simulink model "signalProcess"  (R2016a)
settings: Solver=VariableStepAuto  StartTime=0.0  StopTime=10  RelTol=1e-3
libraries: powerlib x11, powerlib_meascontrol x1
settings Model: Creator=Jasonkay  LastModifiedBy=Jasonkay

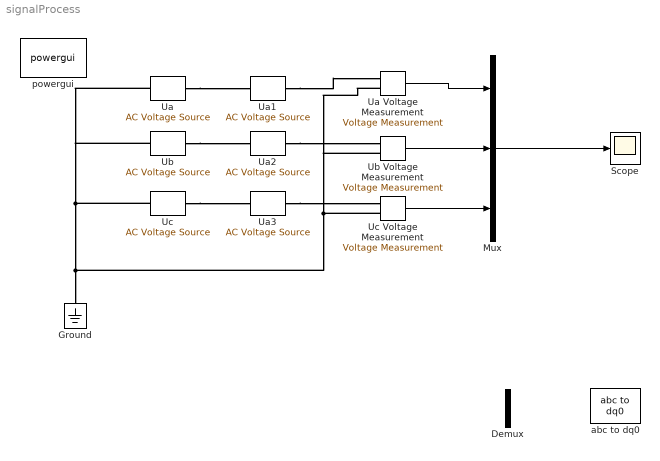
== system signalProcess ==
  Demux : Demux  Outputs=2
  Ground : powerlib/Elements/Ground  LConnTagsString=a
  Mux : Mux  Inputs=3
  Scope : Scope
  Ua : powerlib/Electrical Sources/AC Voltage Source  Amplitude=220 * sqrt(2)  Phase=0  Frequency=50  SampleTime=0  Measurements=None  BusType=swing  Pref=10e3  Qref=0  Qmin=-inf  Qmax=+inf
  Ua Voltage Measurement : powerlib/Measurements/Voltage Measurement  PhasorSimulation=off  OutputType=Complex  PSBequivalent=0
  Ua1 : powerlib/Electrical Sources/AC Voltage Source  Amplitude=20 * sqrt(2)  Phase=0  Frequency=50.1  SampleTime=0  Measurements=None  BusType=swing  Pref=10e3  Qref=0  Qmin=-inf  Qmax=+inf
  Ua2 : powerlib/Electrical Sources/AC Voltage Source  Amplitude=20 * sqrt(2)  Phase=0  Frequency=50.1  SampleTime=0  Measurements=None  BusType=swing  Pref=10e3  Qref=0  Qmin=-inf  Qmax=+inf
  Ua3 : powerlib/Electrical Sources/AC Voltage Source  Amplitude=20 * sqrt(2)  Phase=0  Frequency=50.1  SampleTime=0  Measurements=None  BusType=swing  Pref=10e3  Qref=0  Qmin=-inf  Qmax=+inf
  Ub : powerlib/Electrical Sources/AC Voltage Source  Amplitude=220 * sqrt(2)  Phase=240  Frequency=50  SampleTime=0  Measurements=None  BusType=swing  Pref=10e3  Qref=0  Qmin=-inf  Qmax=+inf
  Ub Voltage Measurement : powerlib/Measurements/Voltage Measurement  PhasorSimulation=off  OutputType=Complex  PSBequivalent=0
  Uc : powerlib/Electrical Sources/AC Voltage Source  Amplitude=220 * sqrt(2)  Phase=120  Frequency=50  SampleTime=0  Measurements=None  BusType=swing  Pref=10e3  Qref=0  Qmin=-inf  Qmax=+inf
  Uc Voltage Measurement : powerlib/Measurements/Voltage Measurement  PhasorSimulation=off  OutputType=Complex  PSBequivalent=0
  abc to dq0 : powerlib_meascontrol/Transformations/abc to dq0  Alignment=90 degrees behind phase A axis
  powergui : powerlib/powergui  Priority=1  SimulationMode=Discrete  SolverType=Tustin/Backward Euler (TBE)  SampleTime=50e-6 / 8 / 10  frequency=60  SPID=off  DisableSnubberDevices=off  DisableRonSwitches=off  DisableVfSwitches=off  SwTol=0  DisplayEquations=off  Interpol=off  ExternalGateDelay=off  methode=off  Ts=10  FunctionMessages=off  echomessages=off  HookPort=off  EnableUseOfTLC=off  x0status=blocks  frequencyindice=50  Pbase=100e6  ErrMax=1e-4  Iterations=50  UnitsV=kV  UnitsW=MW  buscounter=0  RestoreLinks=warning  ResistiveCurrentMeasurement=off  Frange=[0:2:500]  Ylog=off  Xlog=on  ShowGrid=off  save=off  variable=ZData  structure=ScopeData  ZoomFFT=off  StartTime=0  cycles=500  DisplayStyle=2  fundamental=50  FreqAxis=off  MaxFrequency=80  frequencyindicesteady=1  RmsSteady=1  display=off
  wires:
  Ua Voltage Measurement/1 -> Mux/1
  Ub Voltage Measurement/1 -> Mux/2
  Uc Voltage Measurement/1 -> Mux/3
  Mux/1 -> Scope/1
  connections:
  Uc/LConn1 -- Ub/LConn1 -- Ua/LConn1 -- Ub Voltage Measurement/LConn2 -- Ua Voltage Measurement/LConn2 -- Uc Voltage Measurement/LConn2 -- Ground/LConn1
  Ua/RConn1 -- Ua1/LConn1
  Ub/RConn1 -- Ua2/LConn1
  Uc/RConn1 -- Ua3/LConn1
  Ua1/RConn1 -- Ua Voltage Measurement/LConn1
  Ua3/RConn1 -- Uc Voltage Measurement/LConn1
  Ua2/RConn1 -- Ub Voltage Measurement/LConn1
